simulink model "SIMU_systeme_solaire"  (R2019b)
settings: Solver=VariableStepAuto  StartTime=0.0  StopTime=2.16666*365*24*60*60  MaxStep=24*60*60  RelTol=1e-3  EnableMultiTasking=on
model workspace (MATLAB code in the model file):
  | % All values are in SI units.
  | % RGB color vectors are on a normalized 0-1 scale.
  | % Body dimensions are scaled for visualization purposes.
  | % Scaling has no impact on model dynamics.
  | 
  | % Scaling
  | SunScaling = 0.5e2;
  | TerrestrialPlanetScaling = 1.2e3;
  | GasGiantScaling = 2.5e2;
  | 
  | % Sun
  | Sun.M = 1.99e30;
  | Sun.R = 6.96e8*SunScaling;
  | Sun.RGB = [1 0.5 0];
  | Sun.Px = 5.5850e+08;
  | Sun.Py = 5.5850e+08;
  | Sun.Pz = 5.5850e+08;
  | Sun.Vx = -1.4663;
  | Sun.Vy = 11.1238;
  | Sun.Vz = 4.8370;
  | 
  | 
  | % Venus
  | Venus.M = 4.87e24;
  | Venus.R = 6.05e6*TerrestrialPlanetScaling;
  | Venus.RGB = [1 0.9 0];
  | Venus.Px = -1.5041e+10;
  | Venus.Py = 9.7080e+10;
  | Venus.Pz = 4.4635e+10;
  | Venus.Vx = -3.4770e+04;
  | Venus.Vy = -5.5933e+03;
  | Venus.Vz = -316.8994;
  | 
  | % Earth
  | Earth.M = 5.97e24;
  | Earth.R = 6.05e6*TerrestrialPlanetScaling;
  | Earth.RGB = [0.3 0.6 0.8];
  | Earth.Px = -1.1506e+09;
  | Earth.Py = -1.3910e+11;
  | Earth.Pz = -6.0330e+10;
  | Earth.Vx = 2.9288e+04;
  | Earth.Vy = -398.5759;
  | Earth.Vz = -172.5873;
  | 
  | % Mars
  | Mars.M = 6.42e23;
  | Mars.R = 3.39e6*TerrestrialPlanetScaling;
  | Mars.RGB = [0.6 0.2 0.4];
  | Mars.Px = -4.8883e+10;
  | Mars.Py = -1.9686e+11;
  | Mars.Pz = -8.8994e+10;
  | Mars.Vx = 2.4533e+04;
  | Mars.Vy = -2.7622e+03;
  | Mars.Vz = -1.9295e+03;
  | 
  | % Spaceship
  | SP.M = 5.97e24;
  | SP.R = 6.05e6*TerrestrialPlanetScaling;
  | SP.RGB = [0.3 0.6 0.8];
  | SP.Px = -1.1506e+09;
  | SP.Py = -1.3910e+11;
  | SP.Pz = -6.0330e+10;
  | SP.Vx = 2.9288e+04;
  | SP.Vy = -398.5759;
  | SP.Vz = -172.5873;
libraries: nesl_utility x22, sm_lib x11
settings Model: Creator=5578000  LastModifiedBy=alexandrelarroumets
settings DataIOCC: LimitDataPoints=on  ReturnWorkspaceOutputs=off
settings OptimizationCC: LifeSpan=inf
settings DebuggingCC: AllowSymbolicDim=off  SFUnexpectedBacktrackingDiag=warning  SFNoUnconditionalDefaultTransitionDiag=warning  SFExecutionAtInitializationDiag=none  ArithmeticOperatorsInVariantConditions=warning
settings SFSimCC: SimUseLocalCustomCode=off  CustomCodeUndefinedFunction=UseInterfaceOnly
settings RTWCC: RTWUseLocalCustomCode=off
settings CodeAppCC: StateflowObjectComments=on
settings GRTTargetCC: TargetLangStandard=C89/C90 (ANSI)  GeneratePreprocessorConditionals=Disable all
settings ConfigComp: CovMetricSettings=dw  CovHtmlReporting=on  CovSaveCumulativeToWorkspaceVar=on  CovSaveSingleToWorkspaceVar=on  CovExternalEMLEnable=off  CovSFcnEnable=off
settings SimscapeCC: SimscapeNominalValues="[{\"value\":\"10\",\"unit\":\"V\"},{\"value\":\"1\",\"unit\":\"A\"},{\"value\":\"10\",\"unit\":\"N*m\"},{\"value\":\"10\",\"unit\":\"bar\"},{\"value\":\"100\",\"unit\":\"kJ/kg\"},{\"value\":\"1\",\"unit\":\"kW\"},{\"value\":\"300\",\"unit\":\"K\"},{\"value\":\"100\",\"unit\":\"cm^3/s\"},{\"value\":\"1\",\"unit\":\"kN\"},{\"value\":\"1\",\"unit\":\"g/cm^3\"},{\"value\":\"1\",\"unit\":\"l\"},{\"value\":\"1\",\"unit\":\"cm^2\"},{\"value\":\"60\",\"unit\":\"Hz\"}]"  SimscapeLogType=all  SimscapeLogDataHistory=10000
settings ConfigurationSet: Description=SimMechanics 2G
settings ExplorerConfigSet: InternalSimMechanicsExplorerSettings="<ExplorerConfiguration><canonicalview>default</canonicalview><AnimationSetting><BasePlaybackSpeed>8000</BasePlaybackSpeed><PlaybackSpeedFactor>256.0</PlaybackSpeedFactor></AnimationSetting><TilePanel><TileInfo><Tiles Columns=\"1\" Count=\"1\" Rows=\"1\"><Column Weight=\"1\"/><Row Weight=\"1\"/><Tile Height=\"1\" Width=\"1\" X=\"0\" Y=\"0\"/></Tiles></TileInfo><SceneInfo><SceneViewer><BGColor><R>0.60000002384185791</R><G>0.60000002384185791</G><B>0.60000002384185791</B></BGColor><Camera><DoPerspective>off</DoPerspective><Position><X>-2260146179.8719101</X><Y>-124442440268.449829</Y><Z>231075504154.807495</Z></Position><Center><X>13531239847.1738968</X><Y>4166687310.89451599</Y><Z>25540528782.5031738</Z></Center><Up><X>0.639935979456736415</X><Y>0.628344815949277047</Y><Z>0.442340066539780197</Z></Up><ViewLimDist>1</ViewLimDist><YLim>331115561432.217224</YLim><XLim>500382375932.189758</XLim></Camera></SceneViewer></SceneInfo></TilePanel><MechEditorPanel><Cameras/><GfxPanelCameraMap/><VideoCreator><PlaybackSpeedRatio>1.0</PlaybackSpeedRatio><FrameRate>30</FrameRate><VideoFormat>Motion JPEG AVI</VideoFormat><FrameSize>auto</FrameSize></VideoCreator></MechEditorPanel></ExplorerConfiguration>"

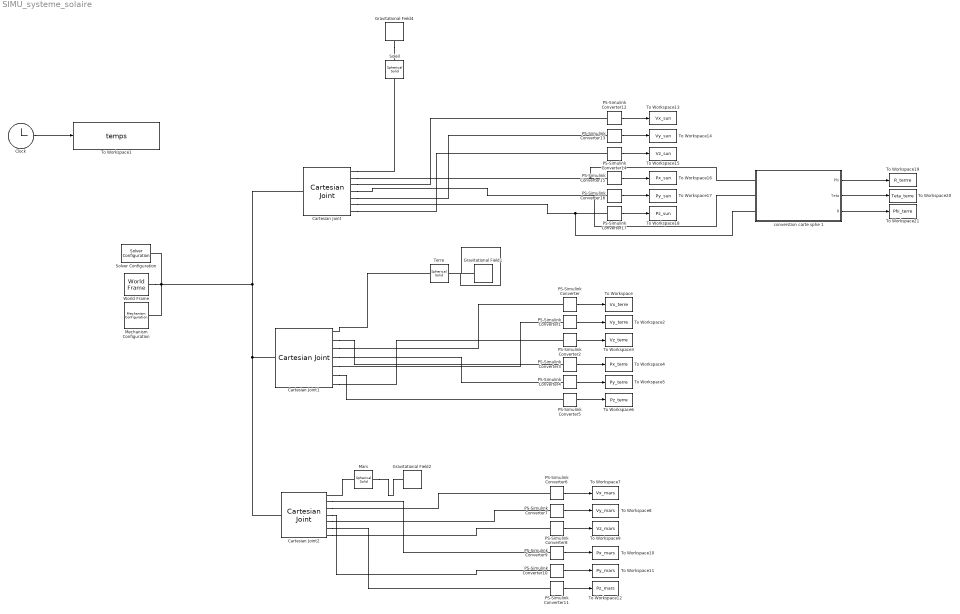
== system SIMU_systeme_solaire ==
  Cartesian Joint : sm_lib/Joints/Cartesian Joint  JointMode=Normal  SenseConstraintForce=off  SenseConstraintForceX=off  SenseConstraintForceY=off  SenseConstraintForceZ=off  SenseConstraintTorque=off  SenseConstraintTorqueX=off  SenseConstraintTorqueY=off  SenseConstraintTorqueZ=off  SenseTotalForce=off  SenseTotalForceX=off  SenseTotalForceY=off  SenseTotalForceZ=off  SenseTotalTorque=off  SenseTotalTorqueX=off  SenseTotalTorqueY=off  SenseTotalTorqueZ=off  CompositeWrenchDir=FollowerOnBase  CompositeWrenchFrame=BaseFrame  PxEquilibriumPosition=0  PxEquilibriumPositionUnits=m  PxSpringStiffness=0  PxSpringStiffnessUnits=N/m  PxDampingCoefficient=0  PxDampingCoefficientUnits=N/(m/s)  PxTorqueActuationMode=NoTorque  PxMotionActuationMode=ComputedMotion  PxSensePosition=on  PxSenseVelocity=on  PxSenseAcceleration=off  PxSenseTorqueForce=off  PxSenseLowerLimitTorqueForce=off  PxSenseUpperLimitTorqueForce=off  PxLowerLimitSpecify=off  PxLowerLimitBound=-1  PxLowerLimitBoundUnits=m  PxLowerLimitStiffness=1e6  PxLowerLimitStiffnessUnits=N/m  PxLowerLimitDamping=1e3  PxLowerLimitDampingUnits=N/(m/s)  PxLowerLimitTransitionRegionWidth=1e-4  PxLowerLimitTransitionRegionWidthUnits=m  PxUpperLimitSpecify=off  PxUpperLimitBound=1  PxUpperLimitBoundUnits=m  PxUpperLimitStiffness=1e6  PxUpperLimitStiffnessUnits=N/m  PxUpperLimitDamping=1e3  PxUpperLimitDampingUnits=N/(m/s)  PxUpperLimitTransitionRegionWidth=1e-4  PxUpperLimitTransitionRegionWidthUnits=m  PxPositionTargetSpecify=on  PxPositionTargetPriority=High  PxPositionTargetValue=Sun.Px  PxPositionTargetValueUnits=m  PxVelocityTargetSpecify=on  PxVelocityTargetPriority=High  PxVelocityTargetValue=Sun.Vx  PxVelocityTargetValueUnits=m/s  PyEquilibriumPosition=0  PyEquilibriumPositionUnits=m  PySpringStiffness=0  PySpringStiffnessUnits=N/m  PyDampingCoefficient=0  PyDampingCoefficientUnits=N/(m/s)  PyTorqueActuationMode=NoTorque  PyMotionActuationMode=ComputedMotion  PySensePosition=on  PySenseVelocity=on  PySenseAcceleration=off  PySenseTorqueForce=off  PySenseLowerLimitTorqueForce=off  PySenseUpperLimitTorqueForce=off  PyLowerLimitSpecify=off  PyLowerLimitBound=-1  PyLowerLimitBoundUnits=m  PyLowerLimitStiffness=1e6  PyLowerLimitStiffnessUnits=N/m  PyLowerLimitDamping=1e3  PyLowerLimitDampingUnits=N/(m/s)  PyLowerLimitTransitionRegionWidth=1e-4  PyLowerLimitTransitionRegionWidthUnits=m  PyUpperLimitSpecify=off  PyUpperLimitBound=1  PyUpperLimitBoundUnits=m  PyUpperLimitStiffness=1e6  PyUpperLimitStiffnessUnits=N/m  PyUpperLimitDamping=1e3  PyUpperLimitDampingUnits=N/(m/s)  PyUpperLimitTransitionRegionWidth=1e-4  PyUpperLimitTransitionRegionWidthUnits=m  PyPositionTargetSpecify=on  PyPositionTargetPriority=High  PyPositionTargetValue=Sun.Py  PyPositionTargetValueUnits=m  PyVelocityTargetSpecify=on  PyVelocityTargetPriority=High  PyVelocityTargetValue=Sun.Vy  PyVelocityTargetValueUnits=m/s  PzEquilibriumPosition=0  PzEquilibriumPositionUnits=m  PzSpringStiffness=0  PzSpringStiffnessUnits=N/m  PzDampingCoefficient=0  PzDampingCoefficientUnits=N/(m/s)  PzTorqueActuationMode=NoTorque  PzMotionActuationMode=ComputedMotion  PzSensePosition=on  PzSenseVelocity=on  PzSenseAcceleration=off  PzSenseTorqueForce=off  PzSenseLowerLimitTorqueForce=off  PzSenseUpperLimitTorqueForce=off  PzLowerLimitSpecify=off  PzLowerLimitBound=-1  PzLowerLimitBoundUnits=m  PzLowerLimitStiffness=1e6  PzLowerLimitStiffnessUnits=N/m  PzLowerLimitDamping=1e3  PzLowerLimitDampingUnits=N/(m/s)  PzLowerLimitTransitionRegionWidth=1e-4  PzLowerLimitTransitionRegionWidthUnits=m  PzUpperLimitSpecify=off  PzUpperLimitBound=1  PzUpperLimitBoundUnits=m  PzUpperLimitStiffness=1e6  PzUpperLimitStiffnessUnits=N/m  PzUpperLimitDamping=1e3  PzUpperLimitDampingUnits=N/(m/s)  PzUpperLimitTransitionRegionWidth=1e-4  PzUpperLimitTransitionRegionWidthUnits=m  PzPositionTargetSpecify=on  PzPositionTargetPriority=High  PzPositionTargetValue=Sun.Pz  PzPositionTargetValueUnits=m  PzVelocityTargetSpecify=on  PzVelocityTargetPriority=High  PzVelocityTargetValue=Sun.Vz  PzVelocityTargetValueUnits=m/s
  Cartesian Joint1 : sm_lib/Joints/Cartesian Joint  JointMode=Normal  SenseConstraintForce=off  SenseConstraintForceX=off  SenseConstraintForceY=off  SenseConstraintForceZ=off  SenseConstraintTorque=off  SenseConstraintTorqueX=off  SenseConstraintTorqueY=off  SenseConstraintTorqueZ=off  SenseTotalForce=off  SenseTotalForceX=off  SenseTotalForceY=off  SenseTotalForceZ=off  SenseTotalTorque=off  SenseTotalTorqueX=off  SenseTotalTorqueY=off  SenseTotalTorqueZ=off  CompositeWrenchDir=FollowerOnBase  CompositeWrenchFrame=BaseFrame  PxEquilibriumPosition=0  PxEquilibriumPositionUnits=m  PxSpringStiffness=0  PxSpringStiffnessUnits=N/m  PxDampingCoefficient=0  PxDampingCoefficientUnits=N/(m/s)  PxTorqueActuationMode=NoTorque  PxMotionActuationMode=ComputedMotion  PxSensePosition=on  PxSenseVelocity=on  PxSenseAcceleration=off  PxSenseTorqueForce=off  PxSenseLowerLimitTorqueForce=off  PxSenseUpperLimitTorqueForce=off  PxLowerLimitSpecify=off  PxLowerLimitBound=-1  PxLowerLimitBoundUnits=m  PxLowerLimitStiffness=1e6  PxLowerLimitStiffnessUnits=N/m  PxLowerLimitDamping=1e3  PxLowerLimitDampingUnits=N/(m/s)  PxLowerLimitTransitionRegionWidth=1e-4  PxLowerLimitTransitionRegionWidthUnits=m  PxUpperLimitSpecify=off  PxUpperLimitBound=1  PxUpperLimitBoundUnits=m  PxUpperLimitStiffness=1e6  PxUpperLimitStiffnessUnits=N/m  PxUpperLimitDamping=1e3  PxUpperLimitDampingUnits=N/(m/s)  PxUpperLimitTransitionRegionWidth=1e-4  PxUpperLimitTransitionRegionWidthUnits=m  PxPositionTargetSpecify=on  PxPositionTargetPriority=High  PxPositionTargetValue=Earth.Px  PxPositionTargetValueUnits=m  PxVelocityTargetSpecify=on  PxVelocityTargetPriority=High  PxVelocityTargetValue=Earth.Vx  PxVelocityTargetValueUnits=m/s  PyEquilibriumPosition=0  PyEquilibriumPositionUnits=m  PySpringStiffness=0  PySpringStiffnessUnits=N/m  PyDampingCoefficient=0  PyDampingCoefficientUnits=N/(m/s)  PyTorqueActuationMode=NoTorque  PyMotionActuationMode=ComputedMotion  PySensePosition=on  PySenseVelocity=on  PySenseAcceleration=off  PySenseTorqueForce=off  PySenseLowerLimitTorqueForce=off  PySenseUpperLimitTorqueForce=off  PyLowerLimitSpecify=off  PyLowerLimitBound=-1  PyLowerLimitBoundUnits=m  PyLowerLimitStiffness=1e6  PyLowerLimitStiffnessUnits=N/m  PyLowerLimitDamping=1e3  PyLowerLimitDampingUnits=N/(m/s)  PyLowerLimitTransitionRegionWidth=1e-4  PyLowerLimitTransitionRegionWidthUnits=m  PyUpperLimitSpecify=off  PyUpperLimitBound=1  PyUpperLimitBoundUnits=m  PyUpperLimitStiffness=1e6  PyUpperLimitStiffnessUnits=N/m  PyUpperLimitDamping=1e3  PyUpperLimitDampingUnits=N/(m/s)  PyUpperLimitTransitionRegionWidth=1e-4  PyUpperLimitTransitionRegionWidthUnits=m  PyPositionTargetSpecify=on  PyPositionTargetPriority=High  PyPositionTargetValue=Earth.Py  PyPositionTargetValueUnits=m  PyVelocityTargetSpecify=on  PyVelocityTargetPriority=High  PyVelocityTargetValue=Earth.Vy  PyVelocityTargetValueUnits=m/s  PzEquilibriumPosition=0  PzEquilibriumPositionUnits=m  PzSpringStiffness=0  PzSpringStiffnessUnits=N/m  PzDampingCoefficient=0  PzDampingCoefficientUnits=N/(m/s)  PzTorqueActuationMode=NoTorque  PzMotionActuationMode=ComputedMotion  PzSensePosition=on  PzSenseVelocity=on  PzSenseAcceleration=off  PzSenseTorqueForce=off  PzSenseLowerLimitTorqueForce=off  PzSenseUpperLimitTorqueForce=off  PzLowerLimitSpecify=off  PzLowerLimitBound=-1  PzLowerLimitBoundUnits=m  PzLowerLimitStiffness=1e6  PzLowerLimitStiffnessUnits=N/m  PzLowerLimitDamping=1e3  PzLowerLimitDampingUnits=N/(m/s)  PzLowerLimitTransitionRegionWidth=1e-4  PzLowerLimitTransitionRegionWidthUnits=m  PzUpperLimitSpecify=off  PzUpperLimitBound=1  PzUpperLimitBoundUnits=m  PzUpperLimitStiffness=1e6  PzUpperLimitStiffnessUnits=N/m  PzUpperLimitDamping=1e3  PzUpperLimitDampingUnits=N/(m/s)  PzUpperLimitTransitionRegionWidth=1e-4  PzUpperLimitTransitionRegionWidthUnits=m  PzPositionTargetSpecify=on  PzPositionTargetPriority=High  PzPositionTargetValue=Earth.Pz  PzPositionTargetValueUnits=m  PzVelocityTargetSpecify=on  PzVelocityTargetPriority=High  PzVelocityTargetValue=Earth.Vz  PzVelocityTargetValueUnits=m/s
  Cartesian Joint2 : sm_lib/Joints/Cartesian Joint  JointMode=Normal  SenseConstraintForce=off  SenseConstraintForceX=off  SenseConstraintForceY=off  SenseConstraintForceZ=off  SenseConstraintTorque=off  SenseConstraintTorqueX=off  SenseConstraintTorqueY=off  SenseConstraintTorqueZ=off  SenseTotalForce=off  SenseTotalForceX=off  SenseTotalForceY=off  SenseTotalForceZ=off  SenseTotalTorque=off  SenseTotalTorqueX=off  SenseTotalTorqueY=off  SenseTotalTorqueZ=off  CompositeWrenchDir=FollowerOnBase  CompositeWrenchFrame=BaseFrame  PxEquilibriumPosition=0  PxEquilibriumPositionUnits=m  PxSpringStiffness=0  PxSpringStiffnessUnits=N/m  PxDampingCoefficient=0  PxDampingCoefficientUnits=N/(m/s)  PxTorqueActuationMode=NoTorque  PxMotionActuationMode=ComputedMotion  PxSensePosition=on  PxSenseVelocity=on  PxSenseAcceleration=off  PxSenseTorqueForce=off  PxSenseLowerLimitTorqueForce=off  PxSenseUpperLimitTorqueForce=off  PxLowerLimitSpecify=off  PxLowerLimitBound=-1  PxLowerLimitBoundUnits=m  PxLowerLimitStiffness=1e6  PxLowerLimitStiffnessUnits=N/m  PxLowerLimitDamping=1e3  PxLowerLimitDampingUnits=N/(m/s)  PxLowerLimitTransitionRegionWidth=1e-4  PxLowerLimitTransitionRegionWidthUnits=m  PxUpperLimitSpecify=off  PxUpperLimitBound=1  PxUpperLimitBoundUnits=m  PxUpperLimitStiffness=1e6  PxUpperLimitStiffnessUnits=N/m  PxUpperLimitDamping=1e3  PxUpperLimitDampingUnits=N/(m/s)  PxUpperLimitTransitionRegionWidth=1e-4  PxUpperLimitTransitionRegionWidthUnits=m  PxPositionTargetSpecify=on  PxPositionTargetPriority=High  PxPositionTargetValue=Mars.Px  PxPositionTargetValueUnits=m  PxVelocityTargetSpecify=on  PxVelocityTargetPriority=High  PxVelocityTargetValue=Mars.Vx  PxVelocityTargetValueUnits=m/s  PyEquilibriumPosition=0  PyEquilibriumPositionUnits=m  PySpringStiffness=0  PySpringStiffnessUnits=N/m  PyDampingCoefficient=0  PyDampingCoefficientUnits=N/(m/s)  PyTorqueActuationMode=NoTorque  PyMotionActuationMode=ComputedMotion  PySensePosition=on  PySenseVelocity=on  PySenseAcceleration=off  PySenseTorqueForce=off  PySenseLowerLimitTorqueForce=off  PySenseUpperLimitTorqueForce=off  PyLowerLimitSpecify=off  PyLowerLimitBound=-1  PyLowerLimitBoundUnits=m  PyLowerLimitStiffness=1e6  PyLowerLimitStiffnessUnits=N/m  PyLowerLimitDamping=1e3  PyLowerLimitDampingUnits=N/(m/s)  PyLowerLimitTransitionRegionWidth=1e-4  PyLowerLimitTransitionRegionWidthUnits=m  PyUpperLimitSpecify=off  PyUpperLimitBound=1  PyUpperLimitBoundUnits=m  PyUpperLimitStiffness=1e6  PyUpperLimitStiffnessUnits=N/m  PyUpperLimitDamping=1e3  PyUpperLimitDampingUnits=N/(m/s)  PyUpperLimitTransitionRegionWidth=1e-4  PyUpperLimitTransitionRegionWidthUnits=m  PyPositionTargetSpecify=on  PyPositionTargetPriority=High  PyPositionTargetValue=Mars.Py  PyPositionTargetValueUnits=m  PyVelocityTargetSpecify=on  PyVelocityTargetPriority=High  PyVelocityTargetValue=Mars.Vy  PyVelocityTargetValueUnits=m/s  PzEquilibriumPosition=0  PzEquilibriumPositionUnits=m  PzSpringStiffness=0  PzSpringStiffnessUnits=N/m  PzDampingCoefficient=0  PzDampingCoefficientUnits=N/(m/s)  PzTorqueActuationMode=NoTorque  PzMotionActuationMode=ComputedMotion  PzSensePosition=on  PzSenseVelocity=on  PzSenseAcceleration=off  PzSenseTorqueForce=off  PzSenseLowerLimitTorqueForce=off  PzSenseUpperLimitTorqueForce=off  PzLowerLimitSpecify=off  PzLowerLimitBound=-1  PzLowerLimitBoundUnits=m  PzLowerLimitStiffness=1e6  PzLowerLimitStiffnessUnits=N/m  PzLowerLimitDamping=1e3  PzLowerLimitDampingUnits=N/(m/s)  PzLowerLimitTransitionRegionWidth=1e-4  PzLowerLimitTransitionRegionWidthUnits=m  PzUpperLimitSpecify=off  PzUpperLimitBound=1  PzUpperLimitBoundUnits=m  PzUpperLimitStiffness=1e6  PzUpperLimitStiffnessUnits=N/m  PzUpperLimitDamping=1e3  PzUpperLimitDampingUnits=N/(m/s)  PzUpperLimitTransitionRegionWidth=1e-4  PzUpperLimitTransitionRegionWidthUnits=m  PzPositionTargetSpecify=on  PzPositionTargetPriority=High  PzPositionTargetValue=Mars.Pz  PzPositionTargetValueUnits=m  PzVelocityTargetSpecify=on  PzVelocityTargetPriority=High  PzVelocityTargetValue=Mars.Vz  PzVelocityTargetValueUnits=m/s
  Clock : Clock
  Gravitational Field1 : sm_lib/Forces and Torques/Gravitational Field  Mass=Earth.M  MassUnits=kg
      settings: SourceProductName=Simscape Multibody  SourceProductBaseCode=MS
  Gravitational Field2 : sm_lib/Forces and Torques/Gravitational Field  Mass=Mars.M  MassUnits=kg
      settings: SourceProductName=Simscape Multibody  SourceProductBaseCode=MS
  Gravitational Field4 : sm_lib/Forces and Torques/Gravitational Field  Mass=Sun.M  MassUnits=kg
      settings: SourceProductName=Simscape Multibody  SourceProductBaseCode=MS
  Mars : sm_lib/Body Elements/Spherical Solid  GraphicAmbientColor=[0.15 0.15 0.15 1.0]  BasedOnType=Mass  CenterOfMass=[0 0 0]  CenterOfMassUnits=m  GraphicDiffuseColor=Mars.RGB  Density=1000  DensityUnits=kg/m^3  DoExposeReferenceFrame=on  GraphicEmissiveColor=[0.0 0.0 0.0 1.0]  ExportEntireGeometry=off  SerializedExposedGeometries=<ExposedGeometries/>  SerializedFrames=<Frames><Frame><Id>Frame1</Id><Value><Name>F1</Name><Origin><Source>ReferenceFrame</Source><FeatureName></FeatureName></Origin><PrimaryAxis><DefinedDirection>+Z</DefinedDirection><Source>ReferenceFrame</Source><SourceDirection>+Z</SourceDirection><FeatureName></FeatureName></PrimaryAxis><SecondaryAxis><DefinedDirection>+X</DefinedDirection><Source>ReferenceFrame</Source><SourceDirection>+X</SourceDirection><FeatureName></FeatureName></SecondaryAxis></Value></Frame></Frames>  MarkerShape=Sphere  MarkerSize=10  GraphicType=FromGeometry  InertiaType=CalculateFromGeometry  Mass=Mars.M  MassUnits=kg  MomentsOfInertia=[1 1 1]  MomentsOfInertiaUnits=kg*m^2  GraphicOpacity=1.0  ProductsOfInertia=[0 0 0]  ProductsOfInertiaUnits=kg*m^2  GraphicShininess=75  GraphicSpecularColor=[0.5 0.5 0.5 1.0]  SphereRadius=Mars.R  SphereRadiusUnits=m  GraphicVisPropType=SimpleVisualProperties
      settings: SourceProductName=Simscape Multibody
  Mechanism Configuration : sm_lib/Utilities/Mechanism Configuration  UniformGravity=None  GravityVector=[0 0 -9.80665]  GravityUnits=m/s^2  LinearizationDelta=0.001
  PS-Simulink Converter{,1..17} (18 alike) : nesl_utility/PS-Simulink Converter  PhysicalDomain=network_engine_domain  SubClassName=ps_output  LeftPortType=input  RightPortType=output  PseudoPeriodic=off  Frequencies=[]  Unit=1  AffineConversion=off
  Soleil : sm_lib/Body Elements/Spherical Solid  GraphicAmbientColor=[0.15 0.15 0.15 1.0]  BasedOnType=Mass  CenterOfMass=[0 0 0]  CenterOfMassUnits=m  GraphicDiffuseColor=Sun.RGB  Density=1000  DensityUnits=kg/m^3  DoExposeReferenceFrame=on  GraphicEmissiveColor=[0.0 0.0 0.0 1.0]  ExportEntireGeometry=off  SerializedExposedGeometries=<ExposedGeometries/>  SerializedFrames=<Frames><Frame><Id>Frame1</Id><Value><Name>F1</Name><Origin><Source>ReferenceFrame</Source><FeatureName></FeatureName></Origin><PrimaryAxis><DefinedDirection>+Z</DefinedDirection><Source>ReferenceFrame</Source><SourceDirection>+Z</SourceDirection><FeatureName></FeatureName></PrimaryAxis><SecondaryAxis><DefinedDirection>+X</DefinedDirection><Source>ReferenceFrame</Source><SourceDirection>+X</SourceDirection><FeatureName></FeatureName></SecondaryAxis></Value></Frame></Frames>  MarkerShape=Sphere  MarkerSize=10  GraphicType=FromGeometry  InertiaType=CalculateFromGeometry  Mass=Sun.M  MassUnits=kg  MomentsOfInertia=[1 1 1]  MomentsOfInertiaUnits=kg*m^2  GraphicOpacity=1.0  ProductsOfInertia=[0 0 0]  ProductsOfInertiaUnits=kg*m^2  GraphicShininess=75  GraphicSpecularColor=[0.5 0.5 0.5 1.0]  SphereRadius=Sun.R  SphereRadiusUnits=m  GraphicVisPropType=SimpleVisualProperties
      settings: SourceProductName=Simscape Multibody
  Solver Configuration : nesl_utility/Solver Configuration  PhysicalDomain=network_engine_domain  SubClassName=solver  LeftPortType=input  RightPortType=generic  Tones=[]  Harmonics=[]  SimulateNoise=off  Profile=off  UseLocalSampling=off  EnableSwitchedLinearOptims=on  FrequencyDomain=off  UseCCode=off  RelTol=0.001  AbsTol=1e-06  MinStep=1e-09  ToWorkspace=off  RevertToSquareIcSolve=off  NumHomotopyIterations=100  PhasorMode=off  PhasorModeNumHarmonics=1  DoDC=off  ResidualTolerance=1e-09  UseLocalSolver=off  LocalSolverChoice=NE_BACKWARD_EULER_ADVANCER  LocalSolverSampleTime=0.001  DoFixedCost=off  MaxNonlinIter=3  MaxModeIter=2  LinearAlgebra=Sparse  EquationFormulation=NE_TIME_EF  DelaysMemoryBudget=1024  AutomaticFiltering=on  FilteringTimeConstant=0.001  PartitionStorageMethod=AS_NEEDED  PartitionMemoryBudget=1024  PartitionMethod=FAST
  Terre : sm_lib/Body Elements/Spherical Solid  GraphicAmbientColor=[0.15 0.15 0.15 1.0]  BasedOnType=Mass  CenterOfMass=[0 0 0]  CenterOfMassUnits=m  GraphicDiffuseColor=Earth.RGB  Density=1000  DensityUnits=kg/m^3  DoExposeReferenceFrame=on  GraphicEmissiveColor=[0.0 0.0 0.0 1.0]  ExportEntireGeometry=off  SerializedExposedGeometries=<ExposedGeometries/>  SerializedFrames=<Frames><Frame><Id>Frame1</Id><Value><Name>F1</Name><Origin><Source>ReferenceFrame</Source><FeatureName></FeatureName></Origin><PrimaryAxis><DefinedDirection>+Z</DefinedDirection><Source>ReferenceFrame</Source><SourceDirection>+Z</SourceDirection><FeatureName></FeatureName></PrimaryAxis><SecondaryAxis><DefinedDirection>+X</DefinedDirection><Source>ReferenceFrame</Source><SourceDirection>+X</SourceDirection><FeatureName></FeatureName></SecondaryAxis></Value></Frame></Frames>  MarkerShape=Sphere  MarkerSize=10  GraphicType=FromGeometry  InertiaType=CalculateFromGeometry  Mass=Earth.M  MassUnits=kg  MomentsOfInertia=[1 1 1]  MomentsOfInertiaUnits=kg*m^2  GraphicOpacity=1.0  ProductsOfInertia=[0 0 0]  ProductsOfInertiaUnits=kg*m^2  GraphicShininess=75  GraphicSpecularColor=[0.5 0.5 0.5 1.0]  SphereRadius=Earth.R  SphereRadiusUnits=m  GraphicVisPropType=SimpleVisualProperties
      settings: SourceProductName=Simscape Multibody
  To Workspace : ToWorkspace  VariableName=Vx_terre  SampleTime=-1
  To Workspace1 : ToWorkspace  VariableName=temps  SampleTime=-1
  To Workspace10 : ToWorkspace  VariableName=Px_mars  SampleTime=-1
  To Workspace11 : ToWorkspace  VariableName=Py_mars  SampleTime=-1
  To Workspace12 : ToWorkspace  VariableName=Pz_mars  SampleTime=-1
  To Workspace13 : ToWorkspace  VariableName=Vx_sun  SampleTime=-1
  To Workspace14 : ToWorkspace  VariableName=Vy_sun  SampleTime=-1
  To Workspace15 : ToWorkspace  VariableName=Vz_sun  SampleTime=-1
  To Workspace16 : ToWorkspace  VariableName=Px_sun  SampleTime=-1
  To Workspace17 : ToWorkspace  VariableName=Py_sun  SampleTime=-1
  To Workspace18 : ToWorkspace  VariableName=Pz_sun  SampleTime=-1
  To Workspace19 : ToWorkspace  VariableName=R_terrre  SampleTime=-1
  To Workspace2 : ToWorkspace  VariableName=Vy_terre  SampleTime=-1
  To Workspace20 : ToWorkspace  VariableName=Teta_terre  SampleTime=-1
  To Workspace21 : ToWorkspace  VariableName=Phi_terre  SampleTime=-1
  To Workspace3 : ToWorkspace  VariableName=Vz_terre  SampleTime=-1
  To Workspace4 : ToWorkspace  VariableName=Px_terre  SampleTime=-1
  To Workspace5 : ToWorkspace  VariableName=Py_terre  SampleTime=-1
  To Workspace6 : ToWorkspace  VariableName=Pz_terre  SampleTime=-1
  To Workspace7 : ToWorkspace  VariableName=Vx_mars  SampleTime=-1
  To Workspace8 : ToWorkspace  VariableName=Vy_mars  SampleTime=-1
  To Workspace9 : ToWorkspace  VariableName=Vz_mars  SampleTime=-1
  World Frame : sm_lib/Frames and Transforms/World Frame
  converstion carte sphe 1 : Subsystem
  wires:
  PS-Simulink Converter/1 -> To Workspace/1
  Clock/1 -> To Workspace1/1
  PS-Simulink Converter1/1 -> To Workspace2/1
  PS-Simulink Converter2/1 -> To Workspace3/1
  PS-Simulink Converter5/1 -> To Workspace6/1
  PS-Simulink Converter4/1 -> To Workspace5/1
  PS-Simulink Converter3/1 -> To Workspace4/1
  PS-Simulink Converter9/1 -> To Workspace10/1
  PS-Simulink Converter10/1 -> To Workspace11/1
  PS-Simulink Converter11/1 -> To Workspace12/1
  PS-Simulink Converter8/1 -> To Workspace9/1
  PS-Simulink Converter7/1 -> To Workspace8/1
  PS-Simulink Converter6/1 -> To Workspace7/1
  PS-Simulink Converter15/1 -> To Workspace16/1
  PS-Simulink Converter16/1 -> To Workspace17/1
  PS-Simulink Converter17/1 -> To Workspace18/1
  PS-Simulink Converter14/1 -> To Workspace15/1
  PS-Simulink Converter13/1 -> To Workspace14/1
  PS-Simulink Converter12/1 -> To Workspace13/1
  converstion carte sphe 1/3("R ") -> To Workspace21/1
  converstion carte sphe 1/2(Teta) -> To Workspace20/1
  converstion carte sphe 1/1(Phi) -> To Workspace19/1
  connections:
  Solver Configuration/RConn1 -- Mechanism Configuration/RConn1 -- World Frame/RConn1 -- Cartesian Joint/LConn1 -- Cartesian Joint2/LConn1 -- Cartesian Joint1/LConn1
  Gravitational Field1/LConn1 -- Terre/LConn1
  Mars/LConn1 -- Gravitational Field2/LConn1
  Gravitational Field4/LConn1 -- Soleil/LConn1
  Cartesian Joint1/RConn7 -- PS-Simulink Converter2/LConn1
  Cartesian Joint/RConn1 -- Soleil/RConn1
  Mars/RConn1 -- Cartesian Joint2/RConn1
  Terre/RConn1 -- Cartesian Joint1/RConn1
  Cartesian Joint2/RConn4 -- PS-Simulink Converter10/LConn1
  Cartesian Joint2/RConn2 -- PS-Simulink Converter9/LConn1
  Cartesian Joint2/RConn3 -- PS-Simulink Converter6/LConn1
  Cartesian Joint1/RConn2 -- PS-Simulink Converter3/LConn1
  Cartesian Joint1/RConn4 -- PS-Simulink Converter4/LConn1
  Cartesian Joint1/RConn6 -- PS-Simulink Converter5/LConn1
  Cartesian Joint2/RConn6 -- PS-Simulink Converter11/LConn1
  Cartesian Joint2/RConn5 -- PS-Simulink Converter7/LConn1
  Cartesian Joint2/RConn7 -- PS-Simulink Converter8/LConn1
  Cartesian Joint/RConn3 -- PS-Simulink Converter12/LConn1
  Cartesian Joint/RConn5 -- PS-Simulink Converter13/LConn1
  Cartesian Joint/RConn7 -- PS-Simulink Converter14/LConn1
  PS-Simulink Converter15/LConn1 -- Cartesian Joint/RConn2 -- converstion carte sphe 1/LConn1
  PS-Simulink Converter16/LConn1 -- Cartesian Joint/RConn4 -- converstion carte sphe 1/LConn2
  PS-Simulink Converter17/LConn1 -- Cartesian Joint/RConn6 -- converstion carte sphe 1/LConn3
  Cartesian Joint1/RConn3 -- PS-Simulink Converter/LConn1
  Cartesian Joint1/RConn5 -- PS-Simulink Converter1/LConn1

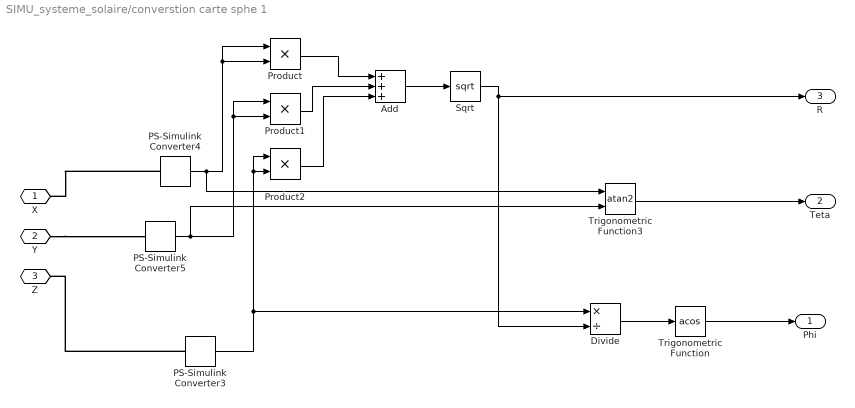
== system SIMU_systeme_solaire/converstion carte sphe 1 ==
  Add : Sum  Inputs=+++
  Divide : Product  Inputs=*/
  PS-Simulink Converter3 : nesl_utility/PS-Simulink Converter  PhysicalDomain=network_engine_domain  SubClassName=ps_output  LeftPortType=input  RightPortType=output  PseudoPeriodic=off  Frequencies=[]  Unit=1  AffineConversion=off
  PS-Simulink Converter4 : nesl_utility/PS-Simulink Converter  PhysicalDomain=network_engine_domain  SubClassName=ps_output  LeftPortType=input  RightPortType=output  PseudoPeriodic=off  Frequencies=[]  Unit=1  AffineConversion=off
  PS-Simulink Converter5 : nesl_utility/PS-Simulink Converter  PhysicalDomain=network_engine_domain  SubClassName=ps_output  LeftPortType=input  RightPortType=output  PseudoPeriodic=off  Frequencies=[]  Unit=1  AffineConversion=off
  Product : Product
  Product1 : Product
  Product2 : Product
  Sqrt : Sqrt  SaturateOnIntegerOverflow=on
  Trigonometric Function : Trigonometry  Operator=acos
  Trigonometric Function3 : Trigonometry  Operator=atan2
  "X " : PMIOPort  Side=Left
  Y : PMIOPort  Port=2  Side=Left
  Z : PMIOPort  Port=3  Side=Left
  Phi : Outport  VectorParamsAs1DForOutWhenUnconnected=off
  Teta : Outport  Port=2  VectorParamsAs1DForOutWhenUnconnected=off
  "R " : Outport  Port=3  VectorParamsAs1DForOutWhenUnconnected=off
  wires:
  Trigonometric Function3/1 -> Teta/1
  PS-Simulink Converter5/1 -> Product1/1, Product1/2, Trigonometric Function3/2
  Trigonometric Function/1 -> Phi/1
  Divide/1 -> Trigonometric Function/1
  Sqrt/1 -> Divide/2, "R "/1
  Add/1 -> Sqrt/1
  Product2/1 -> Add/3
  Product1/1 -> Add/2
  Product/1 -> Add/1
  PS-Simulink Converter4/1 -> Product/1, Product/2, Trigonometric Function3/1
  PS-Simulink Converter3/1 -> Product2/1, Product2/2, Divide/1
  connections:
  PS-Simulink Converter4/LConn1 -- "X "/RConn1
  Y/RConn1 -- PS-Simulink Converter5/LConn1
  PS-Simulink Converter3/LConn1 -- Z/RConn1
